simulink model "Assignment2Sim"  (R2020b)
settings: Solver=ode45  StartTime=0.0  StopTime=70  RelTol=1e-6
values from neighbouring files (symbols this model uses):
  a = 0.4    [Assignment2Mat.m]
  b = 0.4    [Assignment2Mat.m]
  gammaMat = [50 0 ... (first row only)    [Assignment2Mat.m]
  gammaMatD = [50 0 ... (first row only)    [Assignment2Mat.m]
  H1_den = [1 1]    [Assignment2Mat.m]
  H1_num = [1]    [Assignment2Mat.m]
  H2_den = [1 2]    [Assignment2Mat.m]
  H2_num = [2]    [Assignment2Mat.m]
  lambda = 5    [Assignment2Mat.m]
  sineAmp = 10    [Assignment2Mat.m]
  sineFreq = 5/2    (= 2.5)    [Assignment2Mat.m]
  stepAmp = 10    [Assignment2Mat.m]
libraries: simulink x2
settings Model: Creator=Paolo  LastModifiedBy=Paolo

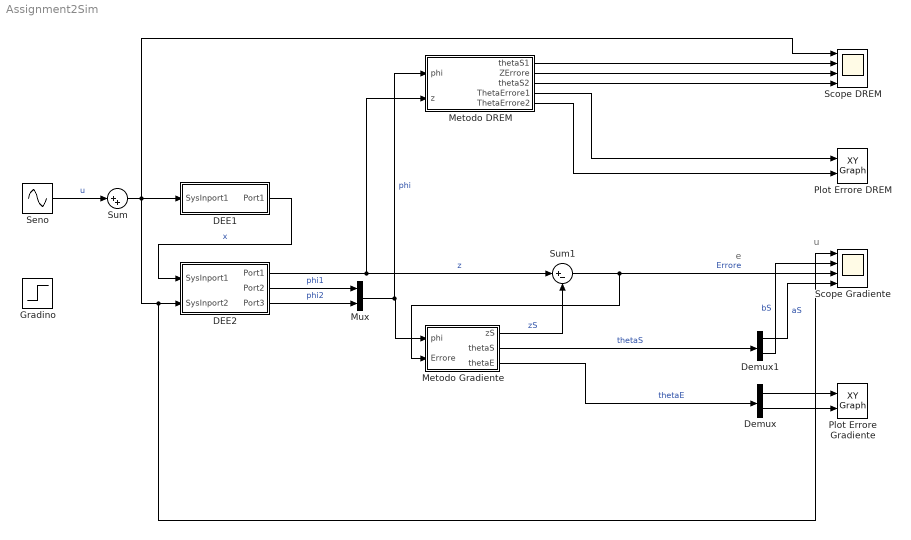
== system Assignment2Sim ==
  note: u
  note: e
  DEE1 : Subsystem  mask(Differential Equation Editor (DEE)){}
      settings: OpenFcn=diffeqed
      mask Display: disp('Sistema')
  DEE2 : Subsystem  mask(Differential Equation Editor (DEE)){}
      settings: OpenFcn=diffeqed
      mask Display: disp('Regressore')
  Demux : Demux  Outputs=2
  Demux1 : Demux  Outputs=2
  Gradino : Step  After=stepAmp  SampleTime=0
  Metodo DREM : Subsystem
  Metodo Gradiente : Subsystem
  Mux : Mux  Inputs=2
  Plot Errore Gradiente : simulink/Sinks/XY Graph  xmin=-0.5  xmax=0.5  ymin=-0.5  ymax=0.5  st=-1
  Plot Errore DREM : simulink/Sinks/XY Graph  xmin=-0.5  xmax=0.5  ymin=-0.5  ymax=0.5  st=-1
  Scope DREM : Scope  NumInputPorts=4
  Scope Gradiente : Scope  NumInputPorts=4
  Seno : Sin  Amplitude=sineAmp  Frequency=sineFreq  SampleTime=0
  Sum : Sum  Inputs=|++
  Sum1 : Sum  Inputs=|+-
  wires:
  DEE1/1(Port1) -> DEE2/1(SysInport1)  "x"
  DEE2/1(Port1) -> Metodo DREM/2(z), Sum1/1  "z"
  DEE2/2(Port2) -> Mux/1  "phi1"
  DEE2/3(Port3) -> Mux/2  "phi2"
  Mux/1 -> Metodo DREM/1(phi), Metodo Gradiente/1(phi)  "phi"
  Metodo Gradiente/1(zS) -> Sum1/2  "zS"
  Sum1/1 -> Scope Gradiente/3, Metodo Gradiente/2(Errore)  "Errore"
  Demux/2 -> Plot Errore Gradiente/2
  Demux/1 -> Plot Errore Gradiente/1
  Metodo Gradiente/3(thetaE) -> Demux/1  "thetaE"
  Metodo Gradiente/2(thetaS) -> Demux1/1  "thetaS"
  Demux1/1 -> Scope Gradiente/4  "aS"
  Demux1/2 -> Scope Gradiente/2  "bS"
  Sum/1 -> Scope DREM/1, Scope Gradiente/1, DEE2/2(SysInport2), DEE1/1(SysInport1)
  Seno/1 -> Sum/1  "u"
  Metodo DREM/4(ThetaErrore1) -> Plot Errore DREM/1
  Metodo DREM/5(ThetaErrore2) -> Plot Errore DREM/2
  Metodo DREM/3(thetaS2) -> Scope DREM/4
  Metodo DREM/2(ZErrore) -> Scope DREM/3
  Metodo DREM/1(thetaS1) -> Scope DREM/2

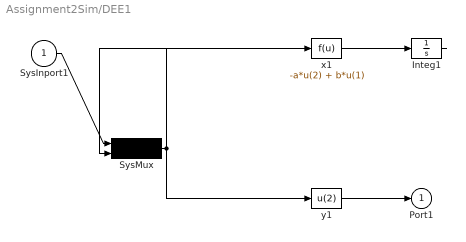
== system Assignment2Sim/DEE1 ==
  SysInport1 : Inport
  Integ1 : Integrator
  SysMux : Mux  Inputs=2
  x1 : Fcn  Expr=-a*u(2) + b*u(1)
  y1 : Fcn  Expr=u(2)
  Port1 : Outport
  wires:
  SysInport1/1 -> SysMux/1
  SysMux/1 -> x1/1, y1/1
  x1/1 -> Integ1/1
  Integ1/1 -> SysMux/2
  y1/1 -> Port1/1

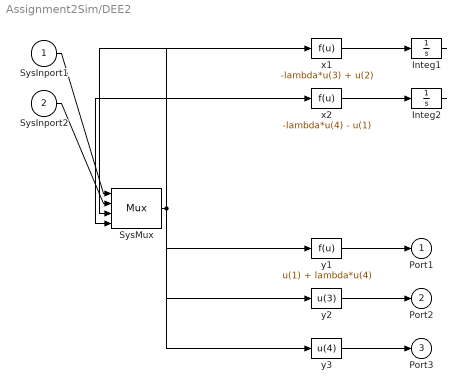
== system Assignment2Sim/DEE2 ==
  SysInport1 : Inport
  SysInport2 : Inport  Port=2
  Integ1 : Integrator
  Integ2 : Integrator
  SysMux : Mux
  x1 : Fcn  Expr=-lambda*u(3) + u(2)
  x2 : Fcn  Expr=-lambda*u(4) - u(1)
  y1 : Fcn  Expr=u(1) + lambda*u(4)
  y2 : Fcn  Expr=u(3)
  y3 : Fcn  Expr=u(4)
  Port1 : Outport
  Port2 : Outport  Port=2
  Port3 : Outport  Port=3
  wires:
  SysInport1/1 -> SysMux/1
  SysInport2/1 -> SysMux/2
  SysMux/1 -> x1/1, x2/1, y1/1, y2/1, y3/1
  x1/1 -> Integ1/1
  Integ1/1 -> SysMux/3
  x2/1 -> Integ2/1
  Integ2/1 -> SysMux/4
  y1/1 -> Port1/1
  y2/1 -> Port2/1
  y3/1 -> Port3/1

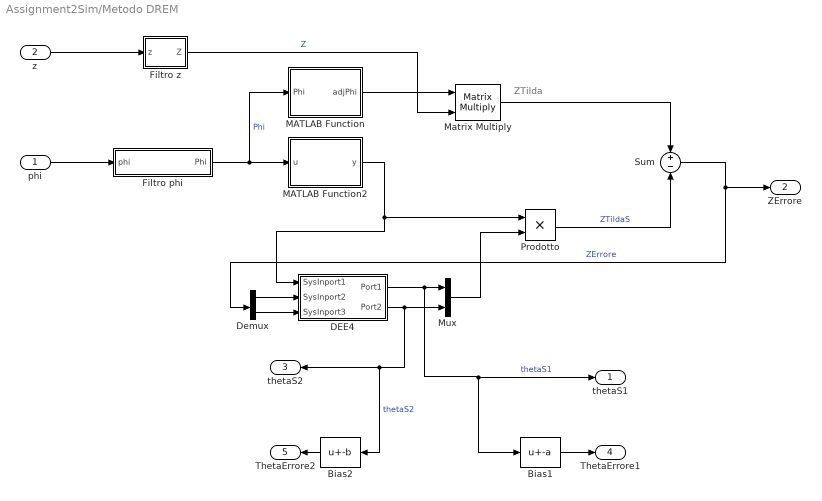
== system Assignment2Sim/Metodo DREM ==
  note: ZTilda
  phi : Inport
  z : Inport  Port=2
  Bias1 : Bias  Bias=-a
  Bias2 : Bias  Bias=-b
  DEE4 : Subsystem  mask(Differential Equation Editor (DEE)){}
      settings: OpenFcn=diffeqed
      mask Display: disp('Stimatore')
  Demux : Demux  Outputs=2
  Filtro phi : Subsystem
  Filtro z : Subsystem
  MATLAB Function : MATLAB Function  TreatAsAtomicUnit=on
  MATLAB Function2 : MATLAB Function  TreatAsAtomicUnit=on
  Matrix Multiply : Product  Multiplication=Matrix(*)
  Mux : Mux  Inputs=2
  Prodotto : Product
  Sum : Sum  Inputs=+|-
  thetaS1 : Outport
  ZErrore : Outport  Port=2
  thetaS2 : Outport  Port=3
  ThetaErrore1 : Outport  Port=4
  ThetaErrore2 : Outport  Port=5
  wires:
  phi/1 -> Filtro phi/1(phi)
  Filtro phi/1(Phi) -> MATLAB Function/1(Phi), MATLAB Function2/1(u)  "Phi"
  z/1 -> Filtro z/1(z)
  Filtro z/1(Z) -> Matrix Multiply/2  "Z"
  MATLAB Function/1(adjPhi) -> Matrix Multiply/1
  Matrix Multiply/1 -> Sum/1
  MATLAB Function2/1(y) -> Prodotto/1, DEE4/1(SysInport1)
  Mux/1 -> Prodotto/2
  DEE4/1(Port1) -> Bias1/1, thetaS1/1, Mux/1  "thetaS1"
  DEE4/2(Port2) -> Bias2/1, thetaS2/1, Mux/2  "thetaS2"
  Prodotto/1 -> Sum/2  "ZTildaS"
  Sum/1 -> ZErrore/1, Demux/1  "ZErrore"
  Demux/2 -> DEE4/3(SysInport3)
  Demux/1 -> DEE4/2(SysInport2)
  Bias1/1 -> ThetaErrore1/1
  Bias2/1 -> ThetaErrore2/1

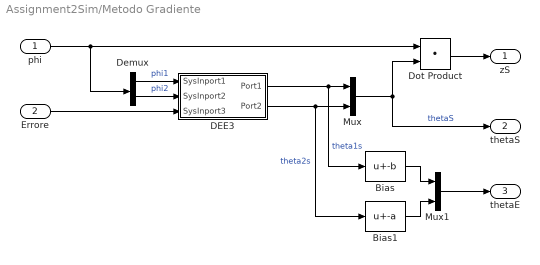
== system Assignment2Sim/Metodo Gradiente ==
  phi : Inport
  Errore : Inport  Port=2
  Bias : Bias  Bias=-b
  Bias1 : Bias  Bias=-a
  DEE3 : Subsystem  mask(Differential Equation Editor (DEE)){}
      settings: OpenFcn=diffeqed
      mask Display: disp('Stimatore')
  Demux : Demux  Outputs=2
  Dot Product : DotProduct  InputSameDT=on  OutDataTypeStr=Inherit: Inherit via internal rule
  Mux : Mux  Inputs=2
  Mux1 : Mux  Inputs=2
  zS : Outport
  thetaS : Outport  Port=2
  thetaE : Outport  Port=3
  wires:
  phi/1 -> Dot Product/1, Demux/1
  Demux/1 -> DEE3/1(SysInport1)  "phi1"
  Demux/2 -> DEE3/2(SysInport2)  "phi2"
  Errore/1 -> DEE3/3(SysInport3)
  DEE3/1(Port1) -> Bias/1, Mux/1  "theta1s"
  DEE3/2(Port2) -> Bias1/1, Mux/2  "theta2s"
  Mux/1 -> thetaS/1, Dot Product/2  "thetaS"
  Dot Product/1 -> zS/1
  Bias/1 -> Mux1/1
  Bias1/1 -> Mux1/2
  Mux1/1 -> thetaE/1

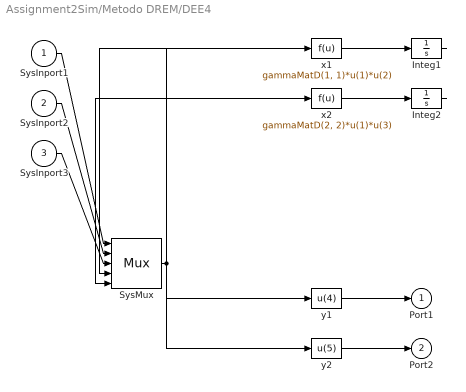
== system Assignment2Sim/Metodo DREM/DEE4 ==
  SysInport1 : Inport
  SysInport2 : Inport  Port=2
  SysInport3 : Inport  Port=3
  Integ1 : Integrator
  Integ2 : Integrator
  SysMux : Mux  Inputs=5
  x1 : Fcn  Expr=gammaMatD(1, 1)*u(1)*u(2)
  x2 : Fcn  Expr=gammaMatD(2, 2)*u(1)*u(3)
  y1 : Fcn  Expr=u(4)
  y2 : Fcn  Expr=u(5)
  Port1 : Outport
  Port2 : Outport  Port=2
  wires:
  SysInport1/1 -> SysMux/1
  SysInport2/1 -> SysMux/2
  SysInport3/1 -> SysMux/3
  SysMux/1 -> x1/1, x2/1, y1/1, y2/1
  x1/1 -> Integ1/1
  Integ1/1 -> SysMux/4
  x2/1 -> Integ2/1
  Integ2/1 -> SysMux/5
  y1/1 -> Port1/1
  y2/1 -> Port2/1

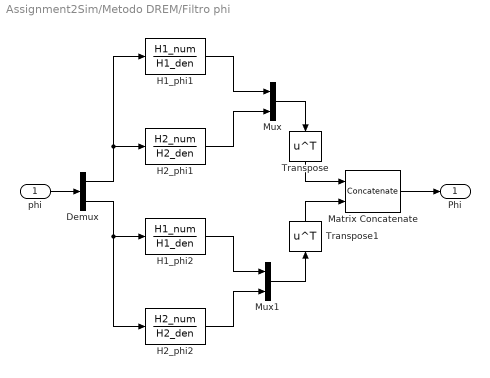
== system Assignment2Sim/Metodo DREM/Filtro phi ==
  phi : Inport
  Demux : Demux  Outputs=2
  H1_phi1 : TransferFcn  Numerator=H1_num  Denominator=H1_den
  H1_phi2 : TransferFcn  Numerator=H1_num  Denominator=H1_den
  H2_phi1 : TransferFcn  Numerator=H2_num  Denominator=H2_den
  H2_phi2 : TransferFcn  Numerator=H2_num  Denominator=H2_den
  Matrix Concatenate : Concatenate  Mode=Multidimensional array
  Mux : Mux  Inputs=2
  Mux1 : Mux  Inputs=2
  Transpose : Math  Operator=transpose  SaturateOnIntegerOverflow=on
  Transpose1 : Math  Operator=transpose  SaturateOnIntegerOverflow=on
  Phi : Outport
  wires:
  Matrix Concatenate/1 -> Phi/1
  phi/1 -> Demux/1
  Demux/1 -> H1_phi1/1, H2_phi1/1
  Demux/2 -> H2_phi2/1, H1_phi2/1
  H1_phi1/1 -> Mux/1
  H2_phi1/1 -> Mux/2
  H1_phi2/1 -> Mux1/1
  H2_phi2/1 -> Mux1/2
  Mux/1 -> Transpose/1
  Mux1/1 -> Transpose1/1
  Transpose/1 -> Matrix Concatenate/1
  Transpose1/1 -> Matrix Concatenate/2

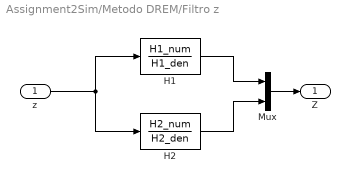
== system Assignment2Sim/Metodo DREM/Filtro z ==
  z : Inport
  H1 : TransferFcn  Numerator=H1_num  Denominator=H1_den
  H2 : TransferFcn  Numerator=H2_num  Denominator=H2_den
  Mux : Mux  Inputs=2
  Z : Outport
  wires:
  Mux/1 -> Z/1
  H1/1 -> Mux/1
  H2/1 -> Mux/2
  z/1 -> H1/1, H2/1

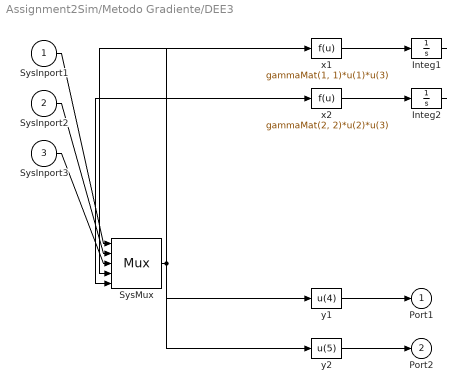
== system Assignment2Sim/Metodo Gradiente/DEE3 ==
  SysInport1 : Inport
  SysInport2 : Inport  Port=2
  SysInport3 : Inport  Port=3
  Integ1 : Integrator
  Integ2 : Integrator
  SysMux : Mux  Inputs=5
  x1 : Fcn  Expr=gammaMat(1, 1)*u(1)*u(3)
  x2 : Fcn  Expr=gammaMat(2, 2)*u(2)*u(3)
  y1 : Fcn  Expr=u(4)
  y2 : Fcn  Expr=u(5)
  Port1 : Outport
  Port2 : Outport  Port=2
  wires:
  SysInport1/1 -> SysMux/1
  SysInport2/1 -> SysMux/2
  SysInport3/1 -> SysMux/3
  SysMux/1 -> x1/1, x2/1, y1/1, y2/1
  x1/1 -> Integ1/1
  Integ1/1 -> SysMux/4
  x2/1 -> Integ2/1
  Integ2/1 -> SysMux/5
  y1/1 -> Port1/1
  y2/1 -> Port2/1

== matlab function Assignment2Sim/Metodo DREM/MATLAB Function2 ==
  data: u input; y output
function y = det(u)
 y =det(u);
end

== matlab function Assignment2Sim/Metodo DREM/MATLAB Function ==
  data: Phi input; adjPhi output
function adjPhi = matAdj(Phi)
    A = zeros(2, 2);
    A(1, 1) = Phi(2, 2);
    A(1, 2) = -Phi(2, 1);
    A(2, 1) = -Phi(1, 2);
    A(2, 2) = Phi(1, 1);
    adjPhi = A;
end
